simulink model "axzblock"  (Simulink 3.00)
settings: Solver=ode45  StartTime=0.0  StopTime=999999  MaxStep=10  RelTol=1e-3  AbsTol=1e-3
settings Model: SaveTime=off  SaveOutput=off

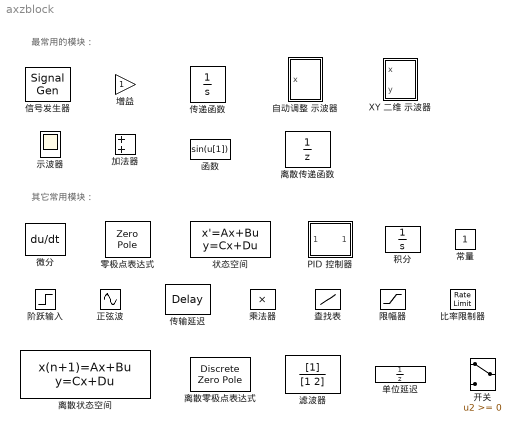
== system axzblock ==
  note: 最常用的模块：
  note: 其它常用模块：
  PID 控制器 : Subsystem  mask(PID Controller){@1=1, @2=1, @3=0}
      mask prompts: @1 "Proportional:"; @2 "Integral"; @3 "Derivative:"
      mask help:
      | Enter expressions for proportional, integral, and derivative terms.
      | P+I/s+Ds
      mask init:
      | P=@1; I=@2; D=@3;
      mask Help: This block implements a PID controller where parameters are entered for the Proportional, Integral and Derivative terms. Unmask this block to see how it works. The derivative term is implemented using a true derivative block.
      mask Display: disp('PID')
  XY 二维 示波器 : Subsystem  mask(XY scope.){@1=-10, @2=10, @3=-10, @4=10}
      mask prompts: @1 "x-min"; @2 "x-max"; @3 "y-min"; @4 "y-max"
      mask help:
      | XY scope using MATLAB graph window.
      | First input is used as time base.
      | Enter plotting ranges.
      mask init:
      | ax = [@1, @2, @3, @4];
      mask Help: This block can be used to explore limit cycles. Look at the m-file sfunxy.m to see how it works.
      mask Display: plot(0,0,100,100,[12,91,91,12,12],[90,90,45,45,90],[51,57,65,75,80,79,75,67,60,54,51,48,42,34,28,27,31,42,51],[71,68,66,66,72,79,83,84,81,77,71,60,54,54,58,65,71,74,71])
  比率限制器 : RateLimiter  RisingSlewLimit=1  FallingSlewLimit=-1
  查找表 : Lookup  InputValues=[-4:5]  OutputValues=rand(1,10)-0.5
  常量 : Constant  Value=1
  乘法器 : Product  Inputs=2  SaturateOnIntegerOverflow=on
  传递函数 : TransferFcn  Numerator=[1]  Denominator=[1 0]
  传输延迟 : TransportDelay  DelayTime=1  InitialInput=0  BufferSize=1024
  单位延迟 : UnitDelay  X0=0  SampleTime=1
  函数 : Fcn  Expr=sin(u[1])
  积分 : Integrator  ExternalReset=none  InitialConditionSource=internal  InitialCondition=0  LimitOutput=off  UpperSaturationLimit=inf  LowerSaturationLimit=-inf  ShowSaturationPort=off  ShowStatePort=off  AbsoluteTolerance=auto
  加法器 : Sum  Inputs=++  SaturateOnIntegerOverflow=on
  阶跃输入 : Step  Time=1  Before=0  After=1  SampleTime=-1
  开关 : Switch  Threshold=0
  离散传递函数 : DiscreteTransferFcn  Numerator=[1]  Denominator=[1 0]  SampleTime=1
  离散零极点表达式 : DiscreteZeroPole  Zeros=[1]  Poles=[0; 0.5]  Gain=[1]  SampleTime=1
  离散状态空间 : DiscreteStateSpace  A=1  B=1  C=1  D=1  X0=0  SampleTime=1
  零极点表达式 : ZeroPole  Zeros=[1]  Poles=[0; -1]  Gain=[1]
  滤波器 : DiscreteFilter  Numerator=[1]  Denominator=[1 2]  SampleTime=1
  示波器 : Scope
      settings: TimeRange=1.000000  YMin=-1.000000  YMax=1.000000  SaveToWorkspace=off  SaveName=ScopeData  DataFormat=Matrix
  微分 : Derivative
  限幅器 : Saturate  UpperLimit=0.5  LowerLimit=-0.5
  信号发生器 : SignalGenerator  WaveForm=sine  Amplitude=1.000000  Frequency=1.000000  Units=rad/sec
  增益 : Gain  Gain=1  SaturateOnIntegerOverflow=on
  正弦波 : Sin  Amplitude=1  Frequency=1  Phase=0  SampleTime=-1
  状态空间 : StateSpace  A=1  B=1  C=1  D=1  X0=0
  自动调整 示波器 : Subsystem  mask(Storage scope.){@1=5, @2=-10, @3=10, @4=200, @5='y-/g--/c-./w:/m*/ro/b+', @6=.1}
      mask prompts: @1 "Initial Time Range:"; @2 "Initial y-min:"; @3 "Initial y-max:"; @4 "Storage pts.:"; @5 "Line type (rgbw-.:xo):"; @6 "Sample time:"
      mask help:
      | Storage scope using MATLAB graph window.
      | Enter plotting ranges and line type.
      mask init:
      | npts = @4; color = @5; ax = [0, @1, @2, @3]; dt=@6;
      mask Help: Uses MATLAB's graph window.\nUse only one block per system.\nLine type must be in quotes.\nSee the M-file sfunyst.m.
      mask Display: plot(0,0,100,100,[83,76,63,52,42,38,28,16,11,84,11,11,11,90,90,11],[75,58,47,54,72,80,84,74,65,65,65,90,40,40,90,90])

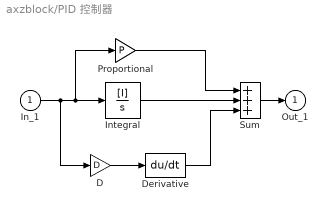
== system axzblock/PID 控制器 ==
  In_1 : Inport  Port=1  PortWidth=-1  SampleTime=-1  DataType=auto
      settings: SignalType=auto
  D : Gain  Gain=D  SaturateOnIntegerOverflow=on
  Derivative : Derivative
  Integral : TransferFcn  Numerator=[I]  Denominator=[1 0]
  Proportional : Gain  Gain=P  SaturateOnIntegerOverflow=on
  Sum : Sum  Inputs=+++  SaturateOnIntegerOverflow=on
  Out_1 : Outport  Port=1
  wires:
  Proportional/1 -> Sum/1
  Integral/1 -> Sum/2
  Derivative/1 -> Sum/3
  In_1/1 -> Integral/1, Proportional/1, D/1
  Sum/1 -> Out_1/1
  D/1 -> Derivative/1

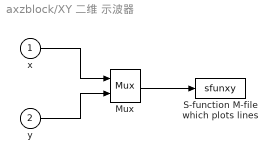
== system axzblock/XY 二维 示波器 ==
  x : Inport  Port=1  PortWidth=-1  SampleTime=-1  DataType=auto
      settings: SignalType=auto
  y : Inport  Port=2  PortWidth=-1  SampleTime=-1  DataType=auto
      settings: SignalType=auto
  Mux : Mux  Inputs=2
      settings: DisplayOption=none
  "S-function M-file which plots lines " : S-Function  FunctionName=sfunxy  Parameters=ax  PortCounts=[]  SFunctionModules=''
  wires:
  Mux/1 -> "S-function M-file which plots lines "/1
  x/1 -> Mux/1
  y/1 -> Mux/2

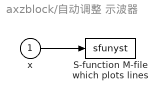
== system axzblock/自动调整 示波器 ==
  x : Inport  Port=1  PortWidth=-1  SampleTime=-1  DataType=auto
      settings: SignalType=auto
  "S-function M-file which plots lines " : S-Function  FunctionName=sfunyst  Parameters=ax, color, npts, dt  PortCounts=[]  SFunctionModules=''
  wires:
  x/1 -> "S-function M-file which plots lines "/1
